simulink model "dft_filter_verificaiton"  (R2021b)
settings: Solver=FixedStepDiscrete  StartTime=0.0  StopTime=6  FixedStep=0.000001  RelTol=1e-3
settings Model: Creator=zqzq_  LastModifiedBy=zqzq_

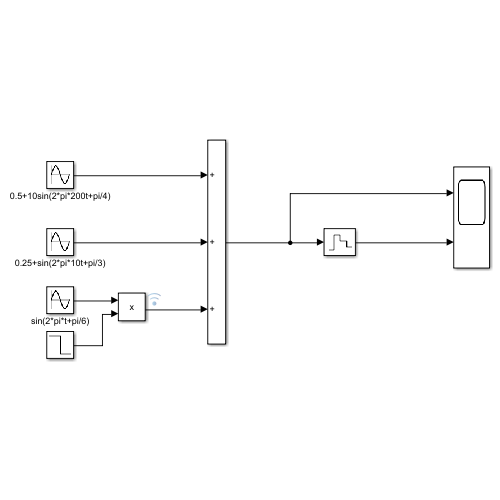
[thumbnail: Simulink's stored preview of the top-level diagram]
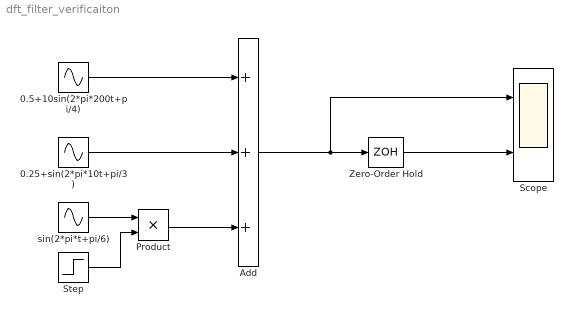
== system dft_filter_verificaiton ==
  0.25+sin(2*pi*10t+pi/3) : Sin  Bias=0.25  Frequency=2*pi*10  Phase=pi/3  SampleTime=0
  0.5+10sin(2*pi*200t+pi/4) : Sin  Amplitude=10  Bias=0.5  Frequency=2*pi*200  Phase=pi/4  SampleTime=0
  Add : Sum  Inputs=+++
  Product : Product
  Scope : Scope  NumInputPorts=2
  Step : Step  Time=3  Before=1  After=0.5  SampleTime=0
  Zero-Order Hold : ZeroOrderHold  SampleTime=0.001
  sin(2*pi*t+pi/6) : Sin  Frequency=2*pi  Phase=pi/6  SampleTime=0
  wires:
  sin(2*pi*t+pi/6)/1 -> Product/1
  Step/1 -> Product/2
  0.5+10sin(2*pi*200t+pi/4)/1 -> Add/1
  0.25+sin(2*pi*10t+pi/3)/1 -> Add/2
  Product/1 -> Add/3
  Add/1 -> Scope/1, Zero-Order Hold/1
  Zero-Order Hold/1 -> Scope/2
